simulink model "AUAV_V3_TestSensors_"  (R2015a)
settings: Solver=FixedStepDiscrete  StartTime=0.0  StopTime=10.0  FixedStep=T  RelTol=1e-3
PreLoadFcn:
  | %T = 0.0025;
  | MavlinkBus;
  | mcuInit;
  | % Baro Altitude Computation
  | % =========================
  | basePressure = 98192.64;
  | baseTemp = 288.215;
  | lapseRate = -0.00198122;
  | baseHeight = 0;
values from neighbouring files (symbols this model uses):
  apSampleTime = 0.01    [mcuInit.m]
  latlong_WP = 1    [mcuInit.m]
  mavlink_attitude_t = Simulink.Bus    [MavlinkBusMarcello.m]
  mavlink_gps_raw_int_t = Simulink.Bus    [MavlinkBus.m]    (also in MavlinkBusMarcello.m)
  mavlink_raw_imu_t = Simulink.Bus    [MavlinkBus.m]    (also in MavlinkBusMarcello.m)
  mavlink_scaled_pressure_t = Simulink.Bus    [MavlinkBus.m]    (also in MavlinkBusMarcello.m)
  mavlink_servo_output_raw_t = Simulink.Bus    [MavlinkBusMarcello.m]
  mavlink_sys_status_t = Simulink.Bus    [MavlinkBus.m]    (also in MavlinkBusMarcello.m)
  T = 0.01    [mcuInit.m]
  Xpoints = [0 0]    [mcuInit.m]
  Ypoints = [0 0]    [mcuInit.m]
  Zpoints = [0 0]    [mcuInit.m]
undefined symbols (not defined in the file or in its folder): A0, A14, A15, A2, A3, A4, A5, A6, accBiasRateLimit, B0, bankCommandLimit, barAdjust, baroCutoff, baroCutTemp, cubeAccelGain16405, cubeGyroGain16405, cubeMagGain16405, D0, D11, D7, D8, daLimit, data, daTrimMax, daTrimMin, deLimit, deTrimMax, deTrimMin, drLimit, drTrimMax, drTrimMin, dtLimit, dtTrimMax, dtTrimMin, F2, F3, G0, G13, G15, gaind, GS_location, gyroBiasRateLimit, IC1max, IPStar, ISA_g, Max, maxAcc, MaxDwnPthStar, maxDynPressure, maxEta, mlParamInterface, ms, OC1max, P112, P125, P127, P16, P20, P21, P30 ... (+26)
undefined symbols (not defined in the file): baroOffset, baroScale, barTGain1, barTGain2, barTMean1, barTMean2, bda, bde, bdr, bdt, bICda, bICde, bICdr, bICdt, derivativesConstant, lowRateSensorCutoff, mainSensorCutoff, mda, mde, mdr, mdt, mICda, mICde, mICdr, mICdt, pitotOffset, pitotScale, pitTGain1, pitTGain2, pitTMean1, pitTMean2, powerOffset, powerScale, pressureSensorCutoff, tempOffset, tempScale, vzCutoff, xCutoff, yCutoff
libraries: MCHP_Blockset x150, simulink x84, SLUGS_Library x31, aerolibconvert2 x6, aerolibutil x4, aerolibtransform2 x3, dspmtrx3 x2, aerolibobsolete x2
(part 6 of 20)

== system AUAV_V3_TestSensors_/Sensor_Data_Adapter ==
  In1 : Inport
  Checks if FixType is 3 [updateSensorMCUState.c]1 : MCHP_Blockset/User Functions/C Function Call  ParseFilesChkbx=on  ListFunctions1=Custom Function  Function1=uint8_t isFixValid (void);  AddHeaderDeclaration=on  Function1Type=when block is updated (default)  FctReturnBlockOut=on  DataCollected="s.chksm=reshape({ '638503-Feb-2015 20:58:10','251913-Sep-2016 12:15:14','1628414-Sep-2016 10:06:29','3862405-Oct-2016 11:19:38','360317-Jun-2016 15:34:16','7114620-Sep-2016 10:38:54','954931-Aug-2016 15:03:40','296127-Sep-2016 09:37:43','268124-Jun-2016 00:23:34','556017-Jun-2016 15:34:16','963217-Jun-2016 15:34:16','1086024-Jun-2016 00:23:34','372414-Sep-2016 14:01:55','998814-Sep-2016 11:55:45','522505-Oct-2016 11:19:36'},1,15);s.File1=reshape({ '  void  newCircBuffer(CBRef cB)','  void  freeCircBuffer(CBRef* cB)','  void  freeCircBuffer(CBRef* cB)',' unsigned int  getLength(CBRef cB)','  int  readHead(CBRef cB)','  int  readTail(CBRef cB)',' unsigned char  peak(CBRef cB)',' unsigned char  readFront(CBRef cB)',' unsigned char  writeBack(CBRef cB, unsigned char data)','  void  makeEmpty(CBRef cB)','  void  printCircBuf(CBRef cB)'},1,11);s.File2=reshape({ '  void  uartBufferInit(void)','  void  __attribute__((__interrupt__, no_auto_psv)) _U4RXInterrupt(void)','  void  getGPSRawData(unsigned char* gpsBuffer)',' unsigned char  isGPSNovatel(void)'},1,4);s.File3=reshape({ '  char  hex2char(char halfhex)','  float  degMinToDeg(unsigned char degrees, float minutes)',' unsigned char  gpsUbloxSeparate(unsigned char* outStream)','  void  gpsUbloxParse(void)','  void  getGpsUbloxMainData(float* data)','  char  gpSmbl(char symbl)',' unsigned char  myTokenizer(char* stringToTokenize, char token, char * returnToken)','  void  parseRMC(unsigned char* stream)','  void  parseGGA(unsigned char* stream)',' unsigned char  getChecksum(unsigned char* sentence, unsigned char size)','  void  gpsDebugMsg(unsigned char buf)'},1,11);s.File4=reshape({ '  void  uartMavlinkBufferInit(void)','  void __attribute__((__interrupt__,__auto_psv__)) _U1RXInterrupt(void)','  uint8_t  isFinite(float s)','  void  InitParameterInterface(void)','  void  protDecodeMavlink(void)','  uint16_t  MissionInterfaceResponse(uint8_t system_id, uint8_t component_id)','  uint16_t  ParameterInterfaceResponse(uint8_t system_id, uint8_t component_id)','  uint16_t  PackHeartBeat(uint8_t system_id, uint8_t component_id)','  uint16_t  PackTextMsg(uint8_t system_id, uint8_t component_id, unsigned char buf)','  uint16_t  PackRawIMU(uint8_t system_id, uint8_t component_id, mavlink_raw_imu_t mlRawIMUData ,uint32_t time_usec)','  uint16_t  PackRawAttitude(uint8_t system_id, uint8_t component_id, mavlink_attitude_t mlAttitudeData ,uint32_t time_usec)','  uint16_t  PackGpsRawInt(uint8_t system_id, uint8_t component_id, mavlink_gps_raw_int_t mlRawGpsDataInt ,uint32_t time_usec)','  uint16_t  PackScaledPressure(uint8_t system_id, uint8_t component_id, mavlink_scaled_pressure_t mlAirData ,uint32_t time_usec)','  uint16_t  PackSysStatus(uint8_t system_id, uint8_t component_id, mavlink_sys_status_t mlSysStatus)','  uint16_t  PackRawServo(uint8_t system_id, uint8_t component_id, mavlink_servo_output_raw_t mlPwmCommands ,uint32_t time_usec)','  uint16_t  HIL_PackRawServo(uint8_t system_id, uint8_t component_id, mavlink_servo_output_raw_t mlPwmCommands ,uint32_t time_usec)','  uint16_t  PackRawRC(uint8_t system_id, uint8_t component_id, mavlink_rc_channels_raw_t mlRC_Commands ,uint32_t time_usec)','  uint16_t  PackVFR_HUD(uint8_t system_id, uint8_t component_id, mavlink_vfr_hud_t mlVfr_hud ,uint32_t time_usec)','  char  sendQGCDebugMessage(const char * dbgMessage, char severity, unsigned char* bytesToAdd, char positionStart)','  void  TxN_Data_OverU1(uint16_t N)','  void  TxN_Data_OverU4(uint16_t N)'},1,21);s.File5=reshape({ '  float  myAtan2(float num, float denom)','  float  myPow(float x, float toTheN)','  float  mySqrt(float x)','  float  myAbs(float x)','  float  myAtan(float x)','  float  myAsin(float x)','  float  mySin(float x)','  float  myCos(float x)','  float  myTan(float x)','  float  myAcos(float x)','  float  myExp(float x)','  void  hugeDelay(void)','  void  smallDelay(void)','  void  tinyDelay(void)','  void  printToUart2(const char *fmt, ...)'},1,15);s.File6=reshape({ '  void  sendTelemetryMavlink(unsigned char* dataOut)','  void  uart2Init(void)','  void  gsRead(unsigned char* gsChunk)','  void  prepareTelemetryMavlink(unsigned char* dataOut)','  void  prepareTelemetryMavlink(unsigned char* dataOut)','  void  sendTelemetryMavlink(unsigned char* dataOut)','  void  copyBufferToDMA1(unsigned char size)','  void  send2GS(unsigned char* protData)','  uint8_t  clearWaypointsFrom(uint8_t startingWp)','  void  addMessageToSpiOut(mavlink_message_t* msg)'},1,10);s.File7={ '  void  populateParameterInterface(void)'};s.File8={ '  void  mavlinkInit(void)'};s.File9=reshape({ '  void  updatePWM(unsigned short * PWMData)','  void  updatePWMTrim(unsigned short PWMData, unsigned char channel)','  void  updateLoad(uint8_t mcuLoad)','  void  updateEuler(float* newEuler)','  void  updatePQR(float* newPQR)',' unsigned char  getHilOnOff(void)','  uint8_t  getLightsOnOff(void)','  uint8_t  getLightsDayNight(void)','  void  updateVISensor(uint16_t* data)','  void  updatePTZ(int16_t* ptz)'},1,10);s.File10=reshape({ '  void  updateRawADCData(int16_t* adcData)','  void  updateAirData(float* airData)','  void  updateLoadData(uint8_t load, uint16_t mvPower)','  void  updateAttitude(float * attitudeData)','  void  getGSLocation(float* altLatLon)','  void  updateTimeStamp(uint32_t timeSt)','  void  updatePosition(float * posData)','  void  updatePilotConsole(uint16_t * pilData)','  void  updateDiagnosticFl(float* diagFl)','  void  updateDiagnosticSh(int16_t* diagSh)','  void  updateBias(float * biasData)','  void  updateSensorData(float* sens)','  uint8_t  isFixValid(void)','  void  updateSensorDiag(float* diag)'},1,14);s.File11=reshape({ '  void  gpsInit(void)','  void  gpsParse(uint8_t* dataStream)','  void  updateStatus(uint8_t* completeMessage)','  void  updatePositionData(uint8_t* completeMessage)','  void  updateVelocityData(uint8_t* completeMessage)','  void  updateTimeData(uint8_t* completeMessage)','  void  getGpsMainData(float* data)','  uint32_t  CRC32Value(int32_t i)','  uint32_t  CalculateBlockCRC32(uint32_t ulCount, uint8_t *ucBuffer)','  uint16_t  charsToUint16(uint8_t* data)','  uint32_t  charsToUint32(uint8_t* data)','  float  charsToFloat(uint8_t* data)','  double  charsToDouble(uint8_t* data)'},1,13);s.File12=reshape({ '  void  getMidLevelCommands(float* commands)',' unsigned char  isApManual(uint16_t failsafe)','  float  getParamIdx(unsigned char idx)','  void  getRangeOfParams(uint8_t startIdx, uint8_t endIdx, float* parameters)','  float  getDynamic(void)','  void  getAttitude(float* attitude)','  void  getXYZ(float* xyz)','  void  getVned(float* xyz)','  uint8_t  getMaxWp(void)',' unsigned char  isWpFly(void)',' unsigned char  isPassthrough(void)','  void  setDiagnosticFloat(float * flValues)','  void  setDiagnosticShort(int16_t* shValues)','  void  getWP(unsigned char idx, float* WPpos)','  void  setLogFloat1(float * flValues)','  void  setLogFloat2(float * flValues)',' unsigned char  getApControlType(void)',' unsigned char  getPassValues(uint8_t* pasVals)','  void  setCurrentCommands(float airSpeed)','  void  getCurrentGPSPos(float* latLonAlt)','  void  setNavLong(float* values)','  void  setNavLat(float* values)','  void  setNavNav(float* values)','  void  getAccels(float * accels)','  void  getAccBias(float * bias)','  void  getRTB(uint8_t* rtb)','  void  getMobileLocation(float* loc)','  uint8_t  getNavMode(void)','  void  getISRLocation(float* loc)','  uint8_t  getISRCameraOption1(void)',' unsigned short  meanFilter5(unsigned short * values)','  uint8_t  justEnabled(uint8_t enableValue, uint8_t index)',' unsigned char  quickSort(unsigned short *arr, char elements)'},1,33);s.File13=reshape({ '  void  hilRead(unsigned char* hilChunk)','  void  hil_getRawRead(short * rawData)','  void  hil_getVned(float* vned)','  void  hil_getEuler(float* euler)','  void  hil_getRates(float* pqr)','  void  hil_getXYZ(float* xyz)',' unsigned int  hil_getTs(void)','  void  protDecodeHil(uint8_t* dataIn)'},1,8);s.File14=reshape({ '  void  cubeInit(void)','  void  getCubeData(short * cubeData)','  void  updateCubeData(void)','  int16_t  averageData(int16_t* theData, uint8_t count)',' unsigned short  write2Cube(unsigned short data2Send)','  short  convert14BitToShort(short wordData)','  short  convert12BitToShort(short wordData)',' unsigned char  isCube16405(void)'},1,8);s.File15=reshape({ '  void  uartMavlinkBufferInit(void)','  uint16_t  PackHeartBeat(uint8_t system_id, uint8_t component_id)','  uint16_t  PackRawServo(uint8_t system_id, uint8_t component_id, mavlink_servo_output_raw_t mlPwmCommands ,uint32_t time_usec)','  uint16_t  HIL_PackRawServo(uint8_t system_id, uint8_t component_id, mavlink_servo_output_raw_t mlPwmCommands ,uint32_t time_usec)','  uint16_t  PackRawRC(uint8_t system_id, uint8_t component_id, mavlink_rc_channels_raw_t mlRC_Commands, uint32_t time_usec)','  uint16_t  PackVFR_HUD(uint8_t system_id, uint8_t component_id, mavlink_vfr_hud_t mlVfr_hud, uint32_t time_usec)','  uint16_t  PackRawIMU(uint8_t system_id, uint8_t component_id, mavlink_raw_imu_t mlRawIMUData ,uint32_t time_usec)','  uint16_t  PackRawAttitude(uint8_t system_id, uint8_t component_id, mavlink_attitude_t mlAttitudeData ,uint32_t time_usec)','  char  sendQGCDebugMessage(const char * dbgMessage, char severity, unsigned char* bytesToAdd, char positionStart)','  uint16_t  PackGpsRawInt(uint8_t system_id, uint8_t component_id, mavlink_gps_raw_int_t mlRawGpsDataInt, uint32_t time_usec)','  uint16_t  PackScaledPressure(uint8_t system_id, uint8_t component_id, mavlink_scaled_pressure_t mlAirData, uint32_t time_usec)','  uint16_t  PackSysStatus(uint8_t system_id, uint8_t component_id, mavlink_sys_status_t mlSysStatus)'},1,12);"  ORDERING=None  SampleTime=.01  MCHP_MASTERLINK=|  PinDigitalInput=[]  PinDigitalOutput=[]  PinAnalogInput=[]
      | AUAV_V3_TestSensors_/Microchip Master
      | AUAV V3 Board
      | Busy Flag on D2 (RA6)
  Data Store Read : DataStoreRead  DataStoreName=GS_INIT_FLAG
  Data Type Conversion : DataTypeConversion  OutDataTypeStr=uint8  SampleTime=0.01
  Enable HIL from Control MCU1 : MCHP_Blockset/Digital IO/Digital Input  Commented=on  PORT=Dynamic Options  PORT_TXT="D   [ 0 : 15 ]"  PIN=[2]  PACK=off  SIMULTANEOUS=off  ORDERING=None  SampleTime=.01  MCHP_PORT={Digital In}{DIN}2:0:D2;  MCHP_MASTERLINK=|
      | AUAV_V3_TestSensors/Microchip Master
      | AUAV V3 Board
      | Busy Flag on D2 (RA6)
  Initialize GS Location : Subsystem
  Logical Operator : Logic  AllPortsSameDT=off  OutDataTypeStr=boolean
  Raw HIL Readings : Subsystem
  Sensor Suite : Subsystem
  Omega (rad/s) : Outport
  Accel (m/s^2) : Outport  Port=2
  Mag (mG) : Outport  Port=3
  Baro Alt (m) : Outport  Port=4
  HIL On? : Outport  Port=5
  GPS : Outport  Port=6
  wires:
  Data Type Conversion/1 -> HIL On?/1
  Sensor Suite/1(Omega (rad/s)) -> Omega (rad/s)/1
  Sensor Suite/2(Accel (m/s^2)) -> Accel (m/s^2)/1
  Sensor Suite/3(Mag (mG)) -> Mag (mG)/1
  Sensor Suite/4(Baro Alt (m)) -> Baro Alt (m)/1
  Sensor Suite/5(GPS) -> GPS/1
  [HIL_FLAG] -> Raw HIL Readings/Enable, Sensor Suite/1(HIL_flag), Data Type Conversion/1
  Raw HIL Readings/1(Raw Msg) -> Sensor Suite/2(Raw HIL)
  In1/1 -> [HIL_FLAG]
  Checks if FixType is 3 [updateSensorMCUState.c]1/1 -> Logical Operator/1
  Data Store Read/1 -> Logical Operator/2
  Logical Operator/1 -> Initialize GS Location/Enable

== system AUAV_V3_TestSensors_/Servo In Out ==
  Bias : Bias  Bias=-round(IC1max/2)
  Bias1 : Bias  Bias=-round(IC1max/2)
  Bias2 : Bias  Bias=+round(IC1max/2)
  Bias3 : Bias  Bias=+round(IC1max/2)
  Constant : Constant  Value=99
  Convert to Microseconds : Subsystem
  Convert to Microseconds1 : Subsystem
  Convert to Microseconds2 : Subsystem
  Data Type Conversion2 : DataTypeConversion  OutDataTypeStr=uint16  ConvertRealWorld=Stored Integer (SI)  RndMeth=Simplest
  Data Type Conversion3 : DataTypeConversion  OutDataTypeStr=uint16  ConvertRealWorld=Stored Integer (SI)  RndMeth=Simplest
  Data Type Conversion4 : DataTypeConversion  OutDataTypeStr=int16  ConvertRealWorld=Stored Integer (SI)  RndMeth=Simplest
  Data Type Conversion5 : DataTypeConversion  OutDataTypeStr=int16  ConvertRealWorld=Stored Integer (SI)  RndMeth=Simplest
  Input Capture RC Receiver1 : MCHP_Blockset/Pulse Input//Output/Input Capture  IntPriority=7  Channel="[1     2     3     4     5     6     7     8]"  Channel_OLD="[1  2  3  4  5  6  7  8]"  PIN_IC1=Dynamic Options  PIN_IC1_TXT=D0 / P64 / Pin[72]  PIN_IC2=Dynamic Options  PIN_IC2_TXT=D8 / P72 / Pin[68]  PIN_IC3=Dynamic Options  PIN_IC3_TXT=D11 / P75 / Pin[71]  PIN_IC4=Dynamic Options  PIN_IC4_TXT=A15 / P31 / Pin[67]  PIN_IC5=Dynamic Options  PIN_IC5_TXT=A5 / P21 / Pin[61]  PIN_IC6=Dynamic Options  PIN_IC6_TXT=A14 / P30 / Pin[66]  PIN_IC7=Dynamic Options  PIN_IC7_TXT=A0 / P16 / Pin[17]  PIN_IC8=Dynamic Options  PIN_IC8_TXT=A0 / P16 / Pin[17]  PIN_IC9=Dynamic Options  PIN_IC9_TXT=A0 / P16 / Pin[17]  PIN_IC10=Dynamic Options  PIN_IC10_TXT=A0 / P16 / Pin[17]  PIN_IC11=Dynamic Options  PIN_IC11_TXT=A0 / P16 / Pin[17]  PIN_IC12=Dynamic Options  PIN_IC12_TXT=A0 / P16 / Pin[17]  PIN_IC13=Dynamic Options  PIN_IC13_TXT=A0 / P16 / Pin[17]  PIN_IC14=Dynamic Options  PIN_IC14_TXT=A0 / P16 / Pin[17]  PIN_IC15=Dynamic Options  PIN_IC15_TXT=A0 / P16 / Pin[17]  PIN_IC16=Dynamic Options  PIN_IC16_TXT=A0 / P16 / Pin[17]  Channel_UP_Down_Periode="[1     1     1     1     1     1     1     1]"  MaxChannel="[0.003   0.003   0.003   0.003   0.003   0.003   0.003   0.003]"  SafeMarge="[0     0     0     0     0     0     0     0]"  MaxChannelValue="2.^[ 14.680  14.680  14.680  14.680  14.680  14.680  14.680  14.680]  =>  [26249  26249  26249  26249  26249  26249  26249  26249]"  ICxmax="[26249  26249  26249  26249  26249  26249  26249  26249]"  Timer="[1  1  1  1  1  1  1  1]"  ChangeDetected="[0     0     0     0     0     0     0     0]"  ChangeDetectedPortRef=3  SampleTime=.02  Status=OK  MCHP_PORT={Input Capture 1}{IC1}6:0:P64;{Input Capture 2}{IC2}6:0:P72;{Input Capture 3}{IC3}6:0:P75;{Input Capture 4}{IC4}6:0:P31;{Input Capture 5}{IC5}6:0:P21;{Input Capture 6}{IC6}6:0:P30;{Input Capture 7}{IC7}6:0:P16;{Input Capture 8}{IC8}6:0:P16;  MCHP_TIMER_REQUEST="{Input Capture 1}{IC1}6:0:1:0:[1  2  3  4  5]:210000;{Input Capture 1}{IC1}6:0:1:0:[1  2  3  4  5]:210000;{Input Capture 1}{IC1}6:0:1:0:[1  2  3  4  5]:210000;{Input Capture 1}{IC1}6:0:1:0:[1  2  3  4  5]:210000;{Input Capture 1}{IC1}6:0:1:0:[1  2  3  4  5]:210000;{Input Capture 1}{IC1}6:0:1:0:[1  2  3  4  5]:210000;{Input Capture 1}{IC1}6:0:1:0:[1  2  3  4  5]:210000;{Input Capture 1}{IC1}6:0:1:0:[1  2  3  4  5]:210000;"  MCHP_TIMER_RESULT=[1 26249.000000000011 ;1 26249.000000000011 ;1 26249.000000000011 ;1 26249.000000000011 ;1 26249.000000000011 ;1 26249.000000000011 ;1 26249.000000000011 ;1 26249.000000000011 ]  MCHP_MASTERLINK=|
      | AUAV_V3_TestSensors/Microchip Master
      | AUAV V3 Board
      | Busy Flag on D2 (RA6)
  Mixing : Subsystem
  Output Compare - HW Drive Servo motor : MCHP_Blockset/Pulse Input//Output/Output Compare - HW  Channel="[1     2]"  Channel_OLD="[1     2]"  PIN_OC1=Dynamic Options  PIN_OC1_TXT=G0 / P112 / Pin[90]  PIN_OC2=Dynamic Options  PIN_OC2_TXT=E0 / P80 / Pin[93]  PIN_OC3=Dynamic Options  PIN_OC3_TXT=D0 / P64 / Pin[72]  PIN_OC4=Dynamic Options  PIN_OC4_TXT=D0 / P64 / Pin[72]  PIN_OC5=Dynamic Options  PIN_OC5_TXT=D0 / P64 / Pin[72]  PIN_OC6=Dynamic Options  PIN_OC6_TXT=D0 / P64 / Pin[72]  PIN_OC7=Dynamic Options  PIN_OC7_TXT=D0 / P64 / Pin[72]  PIN_OC8=Dynamic Options  PIN_OC8_TXT=D0 / P64 / Pin[72]  PIN_OC9=Dynamic Options  PIN_OC9_TXT=D0 / P64 / Pin[72]  PIN_OC10=Dynamic Options  PIN_OC10_TXT=D0 / P64 / Pin[72]  PIN_OC11=Dynamic Options  PIN_OC11_TXT=D0 / P64 / Pin[72]  PIN_OC12=Dynamic Options  PIN_OC12_TXT=D0 / P64 / Pin[72]  PIN_OC13=Dynamic Options  PIN_OC13_TXT=D0 / P64 / Pin[72]  PIN_OC14=Dynamic Options  PIN_OC14_TXT=D0 / P64 / Pin[72]  PIN_OC15=Dynamic Options  PIN_OC15_TXT=D0 / P64 / Pin[72]  PIN_OC16=Dynamic Options  PIN_OC16_TXT=D0 / P64 / Pin[72]  PIN_OCFA=Dynamic Options  PIN_OCFA_TXT=A0 / P16 / Pin[17]  PIN_OCFB=Dynamic Options  PIN_OCFB_TXT=A0 / P16 / Pin[17]  PIN_OCFC=Dynamic Options  PIN_OCFC_TXT=A0 / P16 / Pin[17]  Channel_UP_Down_Periode="[5     5]"  PulseTrig=Single pulse triggered by block execution  InputPeriod=are set to the Max time (constant below)  MaxChannel="[0.003   0.003]"  MaxChannelUnique=.0001  MaxChannelValue="2.^[ 14.680  14.680]  =>  [26249  26249]"  OCxmax="[26249  26249]"  Timer="[1  1]"  SampleTime=.02  MCHP_PORT={Output Compare 1}{OC1}7:1:P112;{Output Compare 2}{OC2}7:1:P80;  MCHP_TIMER_REQUEST="{Output Compare 1}{OC1}7:0:1:0:[1  2  3  4  5]:210000;{Output Compare 1}{OC1}7:0:1:0:[1  2  3  4  5]:210000;"  MCHP_TIMER_RESULT=[1 26249.000000000011 ;1 26249.000000000011 ]  MCHP_MASTERLINK=|
      | AUAV_V3_TestSensors/Microchip Master
      | AUAV V3 Board
      | Busy Flag on D2 (RA6)
  Saturation : Saturate  UpperLimit=OC1max*2.2/3  LowerLimit=OC1max*0.8/3  RndMeth=Simplest
  Saturation1 : Saturate  UpperLimit=OC1max*2.2/3  LowerLimit=OC1max*0.8/3  RndMeth=Simplest
  mlNavigation : DataStoreWrite  DialogController=Simulink.DDGSource  DataStoreName=mlPwmCommands  DataStoreElements=mlPwmCommands.servo1_raw#mlPwmCommands.servo2_raw#mlPwmCommands.servo3_raw#mlPwmCommands.servo4_raw#mlPwmCommands.servo5_raw#mlPwmCommands.servo6_raw#mlPwmCommands.servo7_raw#mlPwmCommands.servo8_raw
  Out1 : Outport
  Out2 : Outport  Port=2
  Out3 : Outport  Port=3
  Out4 : Outport  Port=4
  Out5 : Outport  Port=5
  Out6 : Outport  Port=6
  wires:
  Input Capture RC Receiver1/1 -> Data Type Conversion4/1  "cmd PITCH raw"
  Input Capture RC Receiver1/4 -> Data Type Conversion5/1  "cmd ROLL raw"
  Bias/1 -> Mixing/1(Pitch)
  Bias1/1 -> Mixing/2(Roll)
  Bias2/1 -> Data Type Conversion2/1
  Bias3/1 -> Data Type Conversion3/1
  Saturation1/1 -> Convert to Microseconds1/1(PWM), Output Compare - HW Drive Servo motor/2
  Saturation/1 -> Convert to Microseconds/1(PWM), Output Compare - HW Drive Servo motor/1
  Mixing/2(Cmd Servo Right) -> Bias3/1
  Mixing/1(Cmd Servo Left) -> Bias2/1
  Data Type Conversion4/1 -> Bias/1
  Data Type Conversion5/1 -> Bias1/1
  Data Type Conversion3/1 -> Saturation1/1
  Data Type Conversion2/1 -> Saturation/1
  Input Capture RC Receiver1/2 -> Out1/1
  Input Capture RC Receiver1/3 -> Out2/1
  Input Capture RC Receiver1/5 -> Out3/1
  Input Capture RC Receiver1/6 -> Out4/1
  Input Capture RC Receiver1/7 -> Out5/1
  Input Capture RC Receiver1/8 -> Out6/1
  Constant/1 -> Convert to Microseconds2/1(PWM)
  Convert to Microseconds/1(uS) -> mlNavigation/1
  Convert to Microseconds1/1(uS) -> mlNavigation/2
  Convert to Microseconds2/1(uS) -> mlNavigation/5, mlNavigation/4, mlNavigation/3, mlNavigation/8, mlNavigation/7, mlNavigation/6
